simulink model "Lab2_Sim"  (R2020b)
settings: Solver=VariableStepAuto  StartTime=0.0  StopTime=0.2  RelTol=1e-3
values from neighbouring files (symbols this model uses):
  F = FInt(1 : 4)    [Lab2.m]
  G = inv(sysIO.c*inv(-sysIO.a + sysIO.b*F)*sysIO.b)    [Lab2.m]
settings Model: Creator=Ricardo Wang  LastModifiedBy=DELL
settings SFSimCC: CustomCodeUndefinedFunction=UseInterfaceOnly

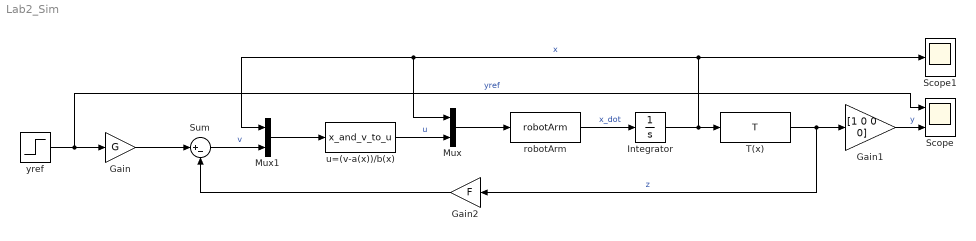
== system Lab2_Sim ==
  Gain : Gain  Gain=G
  Gain1 : Gain  Gain=[1 0 0 0]
  Gain2 : Gain  Gain=F
  Integrator : Integrator
  Mux : Mux  Inputs=2
  Mux1 : Mux  Inputs=2
  Scope : Scope  NumInputPorts=2
  Scope1 : Scope
  Sum : Sum  Inputs=|+-
  T(x) : MATLABFcn  MATLABFcn=T  OutputDimensions=4
  robotArm : MATLABFcn  MATLABFcn=robotArm  OutputDimensions=4
  u=(v-a(x))/b(x) : MATLABFcn  MATLABFcn=x_and_v_to_u  OutputDimensions=1
  yref : Step  SampleTime=0
  wires:
  Integrator/1 -> T(x)/1, Scope1/1, Mux/1, Mux1/1  "x"
  robotArm/1 -> Integrator/1  "x_dot"
  Mux/1 -> robotArm/1
  u=(v-a(x))/b(x)/1 -> Mux/2  "u"
  yref/1 -> Scope/1, Gain/1  "yref"
  Gain/1 -> Sum/1
  T(x)/1 -> Gain2/1, Gain1/1  "z"
  Gain1/1 -> Scope/2  "y"
  Gain2/1 -> Sum/2
  Sum/1 -> Mux1/2  "v"
  Mux1/1 -> u=(v-a(x))/b(x)/1
